simulink model "RZ_EXP1"  (R2020a)
settings: Solver=VariableStepAuto  StartTime=0.0  StopTime=100  RelTol=1e-3
libraries: commrandsrc3 x1
settings Model: Creator=User  LastModifiedBy=Raksha

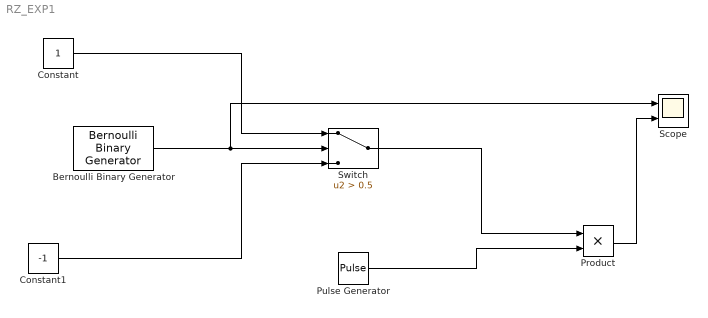
== system RZ_EXP1 ==
  Bernoulli Binary Generator : commrandsrc3/Bernoulli Binary Generator  ProbabilityOfZero=0.5  SeedSource=Auto  Seed=0  SampleTime=1  SamplesPerFrame=1  OutputDataType=double  SimulateUsing=Interpreted execution
  Constant : Constant
  Constant1 : Constant  Value=-1
  Product : Product
  Pulse Generator : DiscretePulseGenerator  PulseType=Time based  Period=1  PulseWidth=50
  Scope : Scope  NumInputPorts=2
  Switch : Switch  Criteria=u2 > Threshold  Threshold=0.5
  wires:
  Constant/1 -> Switch/1
  Bernoulli Binary Generator/1 -> Scope/1, Switch/2
  Constant1/1 -> Switch/3
  Switch/1 -> Product/1
  Pulse Generator/1 -> Product/2
  Product/1 -> Scope/2
